simulink subsystem "ApplicationOpenLoopLowPrio"  (R2024b)
settings: Solver=VariableStepAuto  StartTime=0.0  StopTime=10.0  RelTol=1e-3
settings Model: Creator=The MathWorks, Inc.  LastModifiedBy=The MathWorks, Inc.
settings RTWCC: GPUComputeCapability=3.5

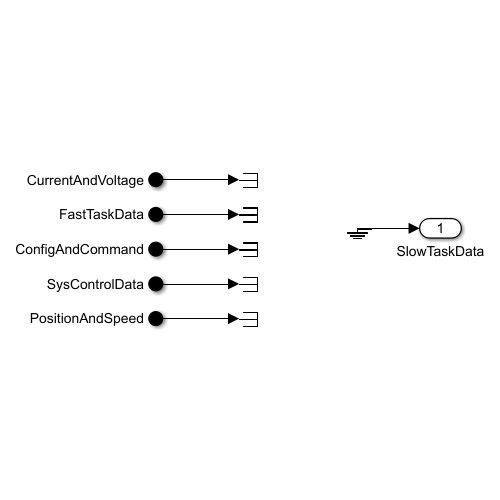
[thumbnail: Simulink's stored preview of the top-level diagram]
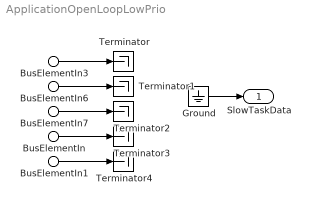
== system ApplicationOpenLoopLowPrio ==
  BusElementIn7 : Inport  PortName=ConfigAndCommand
  BusElementIn3 : Inport  Port=2  PortName=CurrentAndVoltage
  BusElementIn1 : Inport  Port=3  PortName=PositionAndSpeed
  BusElementIn6 : Inport  Port=4  PortName=FastTaskData
  BusElementIn : Inport  Port=5  PortName=SysControlData
  Ground : Ground
  Terminator{,1..4} (5 alike) : Terminator
  SlowTaskData : Outport
  wires:
  BusElementIn3/1 -> Terminator/1
  BusElementIn6/1 -> Terminator1/1
  BusElementIn7/1 -> Terminator2/1
  BusElementIn/1 -> Terminator3/1
  BusElementIn1/1 -> Terminator4/1
  Ground/1 -> SlowTaskData/1
